simulink model "Copy_of_PID_Controller"  (R2023b)
settings: Solver=VariableStepAuto  StartTime=0.0  StopTime=0.02  RelTol=1e-3
libraries: fl_lib x35, nesl_utility x6, ee_lib x1
settings Model: Creator=vkjk4  LastModifiedBy=vkjk4

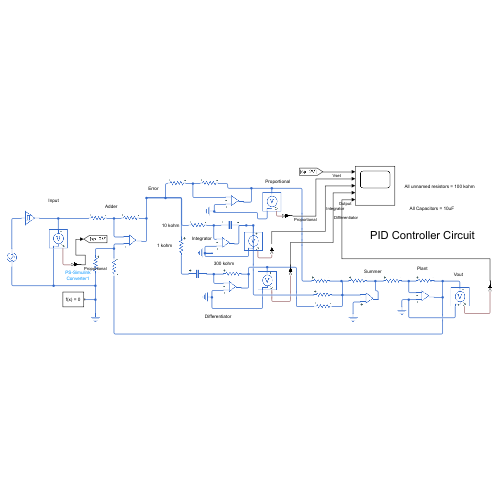
[thumbnail: Simulink's stored preview of the top-level diagram]
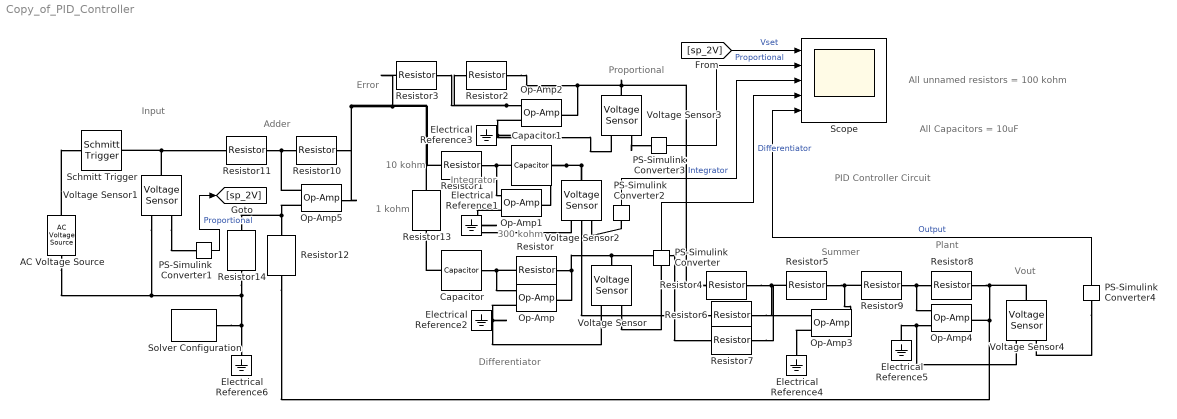
== system Copy_of_PID_Controller ==
  note: All Capacitors = 10uF
  note: All unnamed resistors = 100 kohm
  note: PID Controller Circuit
  note: 300 kohm
  note: 1 kohm
  note: 10 kohm
  note: Input
  note: Adder
  note: Plant
  note: Summer
  note: Differentiator
  note: Integrator
  note: Proportional
  note: Error
  note: Vout
  AC Voltage Source : fl_lib/Electrical/Electrical Sources/AC Voltage Source  amp=3 V  shift=0 deg  frequency=50 Hz  omega=0 rad/s
  Capacitor : fl_lib/Electrical/Electrical Elements/Capacitor  c=10e-6 F  r=1e-6 Ohm  g=0 1/Ohm  i_specify=off  i_priority=None  i=0 A  i_nominal_specify=off  i_nominal_unit=A  i_nominal_value=1  v_specify=off  v_priority=None  v=0 V  v_nominal_specify=off  v_nominal_unit=V  v_nominal_value=1  vc_specify=off  vc_priority=High  vc=0 V  vc_nominal_specify=off  vc_nominal_unit=V  vc_nominal_value=1
  Capacitor1 : fl_lib/Electrical/Electrical Elements/Capacitor  c=10e-6 F  r=1e-6 Ohm  g=0 1/Ohm  i_specify=off  i_priority=None  i=0 A  i_nominal_specify=off  i_nominal_unit=A  i_nominal_value=1  v_specify=off  v_priority=None  v=0 V  v_nominal_specify=off  v_nominal_unit=V  v_nominal_value=1  vc_specify=off  vc_priority=High  vc=0 V  vc_nominal_specify=off  vc_nominal_unit=V  vc_nominal_value=1
  Electrical Reference{1..6} (6 alike) : fl_lib/Electrical/Electrical Elements/Electrical Reference
  Op-Amp{,1..5} (6 alike) : fl_lib/Electrical/Electrical Elements/Op-Amp  outI_specify=off  outI_priority=None  outI=0 A  outI_nominal_specify=off  outI_nominal_unit=A  outI_nominal_value=1
  PS-Simulink Converter{,1..4} (5 alike) : nesl_utility/PS-Simulink Converter  PhysicalDomain=network_engine_domain  SubClassName=ps_output  LeftPortType=input  RightPortType=output  PseudoPeriodic=off  Frequencies=[]  VectorFormat=inherit  Unit=inherit  AffineConversion=off
  Resistor : fl_lib/Electrical/Electrical Elements/Resistor  R=300 kOhm  i_specify=off  i_priority=None  i=0 A  i_nominal_specify=off  i_nominal_unit=A  i_nominal_value=1  v_specify=off  v_priority=None  v=0 V  v_nominal_specify=off  v_nominal_unit=V  v_nominal_value=1
  Resistor1 : fl_lib/Electrical/Electrical Elements/Resistor  R=10 kOhm  i_specify=off  i_priority=None  i=0 A  i_nominal_specify=off  i_nominal_unit=A  i_nominal_value=1  v_specify=off  v_priority=None  v=0 V  v_nominal_specify=off  v_nominal_unit=V  v_nominal_value=1
  Resistor{2..5,7,9..12,14} (10 alike) : fl_lib/Electrical/Electrical Elements/Resistor  R=100 kOhm  i_specify=off  i_priority=None  i=0 A  i_nominal_specify=off  i_nominal_unit=A  i_nominal_value=1  v_specify=off  v_priority=None  v=0 V  v_nominal_specify=off  v_nominal_unit=V  v_nominal_value=1
  Resistor13 : fl_lib/Electrical/Electrical Elements/Resistor  R=1 kOhm  i_specify=off  i_priority=None  i=0 A  i_nominal_specify=off  i_nominal_unit=A  i_nominal_value=1  v_specify=off  v_priority=None  v=0 V  v_nominal_specify=off  v_nominal_unit=V  v_nominal_value=1
  Resistor6 : fl_lib/Electrical/Electrical Elements/Resistor  R=100 Ohm  i_specify=off  i_priority=None  i=0 A  i_nominal_specify=off  i_nominal_unit=A  i_nominal_value=1  v_specify=off  v_priority=None  v=0 V  v_nominal_specify=off  v_nominal_unit=V  v_nominal_value=1
  Resistor8 : fl_lib/Electrical/Electrical Elements/Resistor  R=50 kOhm  i_specify=off  i_priority=None  i=0 A  i_nominal_specify=off  i_nominal_unit=A  i_nominal_value=1  v_specify=off  v_priority=None  v=0 V  v_nominal_specify=off  v_nominal_unit=V  v_nominal_value=1
  Schmitt Trigger : ee_lib/Integrated Circuits/Logic/Schmitt Trigger  V_IL=0 V  V_IH=2 V  C_IN=5 pF  output_type=ee.enum.ic.outputType.linear  V_OL=0 V  V_OH=2 V  V_CC=5 V  V_meas=5 V  R_OUT=25 Ohm  R_OH=[25, 250] Ohm  I_OH=63 mA  R_OL=[30, 800] Ohm  I_OL=-45 mA  Delay=25 ns  Ron=5 Ohm  Vf=0.6 V  output_state=ee.enum.ic.initialState.low
      settings: InternalSimscapePortConfiguration="{\"Bottom\":[],\"Left\":[{\"id\":\"A\",\"label\":\"\",\"type\":\"foundation.electrical.electrical\"}],\"Right\":[{\"id\":\"J\",\"label\":\"\",\"type\":\"foundation.electrical.electrical\"}],\"Top\":[]}"
  Scope : Scope  NumInputPorts=5
  Solver Configuration : nesl_utility/Solver Configuration  PhysicalDomain=network_engine_domain  SubClassName=solver  LeftPortType=input  RightPortType=generic  Tones=[]  Harmonics=[]  SimulateNoise=off  Profile=off  UseLocalSampling=off  EnableSwitchedLinearOptims=on  FrequencyDomain=off  UseCCode=off  RelTol=0.001  AbsTol=0.001  MinStep=1e-09  ToWorkspace=off  RevertToSquareIcSolve=off  NumHomotopyIterations=100  PhasorMode=off  PhasorModeNumHarmonics=1  ConsistencySolver=NEWTON_XTOL_AFTER_FTOL  IndexReductionMethod=DerivativeReplacement  DoDC=off  ResidualTolerance=1e-09  ConsistencyTolSource=GLOBAL  ConsistencyAbsTol=0.001  ConsistencyRelTol=0.001  ConsistencyTolFactor=0.001  UseLocalSolver=off  LocalSolverChoice=NE_BACKWARD_EULER_ADVANCER  ResolveIndetEquations=on  FunctionEvalNumThread=1  LocalSolverSampleTime=0.001  DoFixedCost=off  MaxNonlinIter=3  MaxModeIter=2  ComputeImpulses=off  ImpulseIterations=2  LinearAlgebra=auto  LinearAlgebraNumThread=0  EquationFormulation=NE_TIME_EF  DelaysMemoryBudget=1024  AutomaticFiltering=on  FilteringTimeConstant=0.001  PartitionStorageMethod=AS_NEEDED  PartitionMemoryBudget=1024  PartitionMethod=ROBUST  MultibodyUseLocalSolver=off  MultibodyLocalSolverChoice=ODE1  MultibodyLocalSolverSampleTime=0.001
  Voltage Sensor{,1..4} (5 alike) : fl_lib/Electrical/Electrical Sensors/Voltage Sensor
  wires:
  PS-Simulink Converter/1 -> Scope/4  "Differentiator"
  PS-Simulink Converter2/1 -> Scope/3  "Integrator"
  PS-Simulink Converter3/1 -> Scope/2  "Proportional"
  PS-Simulink Converter4/1 -> Scope/5  "Output"
  [sp_2V] -> Scope/1  "Vset"
  PS-Simulink Converter1/1 -> [sp_2V]  "Proportional"
  connections:
  Op-Amp/LConn1 -- Electrical Reference2/LConn1 -- Voltage Sensor/RConn2
  Capacitor/RConn1 -- Resistor/LConn1 -- Op-Amp/LConn2
  Resistor/RConn1 -- Resistor7/LConn1 -- Voltage Sensor/LConn1 -- Op-Amp/RConn1
  Voltage Sensor/RConn1 -- PS-Simulink Converter/LConn1
  Resistor1/LConn1 -- Resistor10/RConn1 -- Op-Amp5/RConn1 -- Resistor13/LConn1 -- Resistor3/LConn1
  Capacitor1/LConn1 -- Resistor1/RConn1 -- Op-Amp1/LConn2
  Voltage Sensor2/RConn1 -- PS-Simulink Converter2/LConn1
  Op-Amp2/LConn1 -- Electrical Reference3/LConn1 -- Voltage Sensor3/RConn2
  Voltage Sensor3/LConn1 -- Resistor4/LConn1 -- Resistor2/RConn1 -- Op-Amp2/RConn1
  Op-Amp2/LConn2 -- Resistor2/LConn1 -- Resistor3/RConn1
  Voltage Sensor3/RConn1 -- PS-Simulink Converter3/LConn1
  AC Voltage Source/RConn1 -- Voltage Sensor1/RConn2 -- Solver Configuration/RConn1 -- Electrical Reference6/LConn1 -- Resistor14/RConn1
  Op-Amp1/LConn1 -- Electrical Reference1/LConn1 -- Voltage Sensor2/RConn2
  Resistor4/RConn1 -- Resistor6/RConn1 -- Resistor7/RConn1 -- Op-Amp3/LConn2 -- Resistor5/LConn1
  Op-Amp3/LConn1 -- Electrical Reference4/LConn1
  Voltage Sensor2/LConn1 -- Resistor6/LConn1 -- Capacitor1/RConn1 -- Op-Amp1/RConn1
  PS-Simulink Converter4/LConn1 -- Voltage Sensor4/RConn1
  Resistor9/RConn1 -- Op-Amp4/LConn2 -- Resistor8/LConn1
  Resistor9/LConn1 -- Resistor5/RConn1 -- Op-Amp3/RConn1
  Electrical Reference5/LConn1 -- Voltage Sensor4/RConn2 -- Op-Amp4/LConn1
  Resistor11/RConn1 -- Op-Amp5/LConn2 -- Resistor10/LConn1
  Voltage Sensor4/LConn1 -- Resistor8/RConn1 -- Resistor12/RConn1 -- Op-Amp4/RConn1
  Capacitor/LConn1 -- Resistor13/RConn1
  Op-Amp5/LConn1 -- Resistor14/LConn1 -- Resistor12/LConn1
  Voltage Sensor1/RConn1 -- PS-Simulink Converter1/LConn1
  Voltage Sensor1/LConn1 -- Schmitt Trigger/RConn1 -- Resistor11/LConn1
  AC Voltage Source/LConn1 -- Schmitt Trigger/LConn1
